simulink model "untitled"  (R2023b)
settings: Solver=VariableStepAuto  StartTime=0.0  StopTime=1  RelTol=1e-3
libraries: commdigbbndpm3 x2, dspfdesign x2, commchan3 x1, commsink2 x1, commrandsrc3 x1
settings Model: Creator=Bunakov Egor  LastModifiedBy=Bunakov Egor

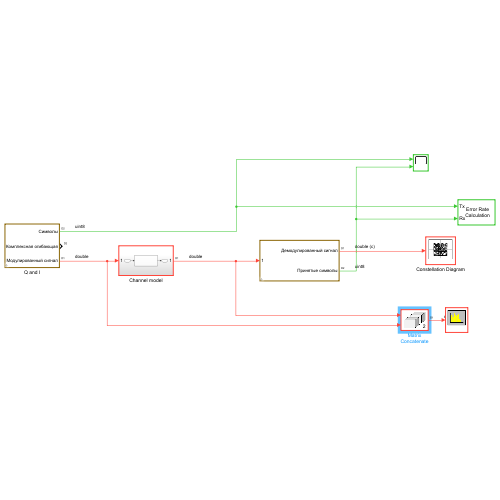
[thumbnail: Simulink's stored preview of the top-level diagram]
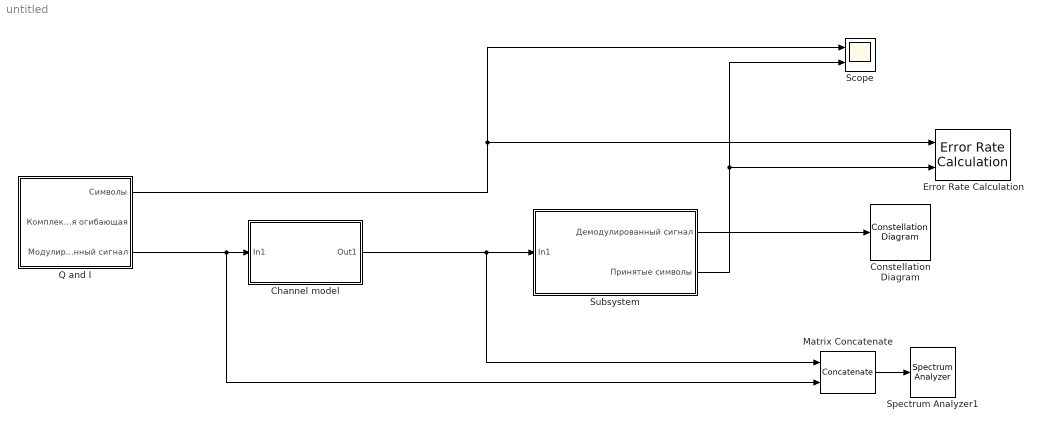
== system untitled ==
  Channel model : Subsystem
  Constellation Diagram : ConstellationDiagram  WindowPosition=[220.000000,9.000000,600.000000,600.000000,]  ScopeFrameLocation=window  ShowTrajectory=on
  Error Rate Calculation : commsink2/Error Rate Calculation  N=0  st_delay=0  cp_mode=Entire frame  subframe=[]  PMode=Workspace  WsName=ErrorVec  RsMode2=off  stop=off  numErr=100  maxBits=1e6
      settings: LibrarySourceBlock=|
      | commhdlsink/Error Rate
      | Calculation
  Matrix Concatenate : Concatenate  Mode=Multidimensional array  ConcatenateDimension=2
  Q and I : Subsystem  mask{CarrierFrequency=10000, SamplingFrequency=100000, SymbolRate=1000}
      mask prompts: CarrierFrequency "Частота несущей"; SamplingFrequency "Частота отрисовки синуса"; SymbolRate "Частота прихода данных"
  Scope : Scope  NumInputPorts=2
  Spectrum Analyzer1 : SpectrumAnalyzer  WindowPosition=[567.000000,192.000000,800.000000,500.000000,]  ScopeFrameLocation=window  YLimits=[-52.67376083,21.22078734]
  Subsystem : Subsystem  mask{SymbolRate=1000, CarrierFrequency=10000, SamplingFrequency=100000}
      mask prompts: SymbolRate "Частота выхода данных"; CarrierFrequency "Частота несущей"; SamplingFrequency "Частота отрисовки синуса"
  wires:
  Q and I/3(Модулированный сигнал) -> Matrix Concatenate/2, Channel model/1(In1)
  Channel model/1(Out1) -> Matrix Concatenate/1, Subsystem/1(In1)
  Subsystem/1(Демодулированный сигнал) -> Constellation Diagram/1
  Q and I/1(Символы) -> Error Rate Calculation/1, Scope/1
  Subsystem/2(Принятые символы) -> Error Rate Calculation/2, Scope/2
  Matrix Concatenate/1 -> Spectrum Analyzer1/1

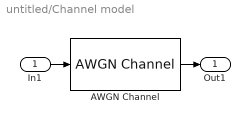
== system untitled/Channel model ==
  In1 : Inport
  AWGN Channel : commchan3/AWGN Channel  LegacyMode=off  NoiseMethod="Signal to noise ratio  (SNR)"  noiseMode="Signal to noise ratio  (SNR)"  EbNo=10  EsNo=10  SNR=100  BitsPerSymbol=1  SignalPower=1  SamplesPerSymbol=1  SymbolPeriod=1  VarianceSource=Parameter  Variance=1  RandomStream=Global stream  Seed=67  SimulateUsing=Code generation
  Out1 : Outport
  wires:
  In1/1 -> AWGN Channel/1
  AWGN Channel/1 -> Out1/1

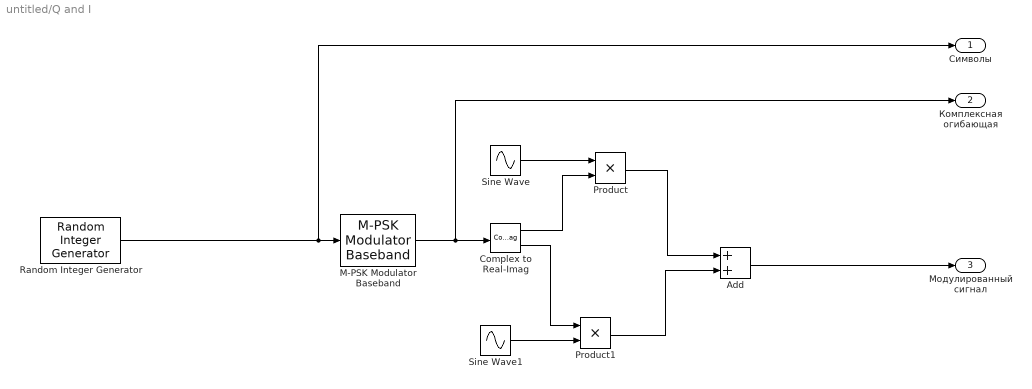
== system untitled/Q and I ==
  Add : Sum
  Complex to Real-Imag : ComplexToRealImag
  M-PSK Modulator Baseband : commdigbbndpm3/M-PSK Modulator Baseband  M=4  InType=Integer  Enc=Gray  Mapping=[0:7]  Ph=pi/4  outDtype=double  outWordLen=16  outUDDataType=sfix(16)  outFracLenMode=Best precision  outFracLen=15  outDataTypeStr=double  outLastDataTypeStr=double
      settings: LibrarySourceBlock=|
      | commhdldigbbndpm/M-PSK
      | Modulator
      | Baseband
  Product : Product
  Product1 : Product
  Random Integer Generator : commrandsrc3/Random Integer Generator  SetSize=4  SeedSource=Auto  Seed=0  SampleTime=1/SymbolRate  SamplesPerFrame=1  OutputDataType=uint8  SimulateUsing=Interpreted execution
  Sine Wave : Sin  Frequency=2*pi*CarrierFrequency  SampleTime=1/SamplingFrequency
  Sine Wave1 : Sin  Frequency=2*pi*CarrierFrequency  Phase=pi/2  SampleTime=1/SamplingFrequency
  Символы : Outport
  Комплексная огибающая : Outport  Port=2
  Модулированный сигнал : Outport  Port=3
  wires:
  Random Integer Generator/1 -> M-PSK Modulator Baseband/1, Символы/1
  M-PSK Modulator Baseband/1 -> Комплексная огибающая/1, Complex to Real-Imag/1
  Sine Wave/1 -> Product/1
  Complex to Real-Imag/1 -> Product/2
  Sine Wave1/1 -> Product1/2
  Complex to Real-Imag/2 -> Product1/1
  Product1/1 -> Add/2
  Product/1 -> Add/1
  Add/1 -> Модулированный сигнал/1

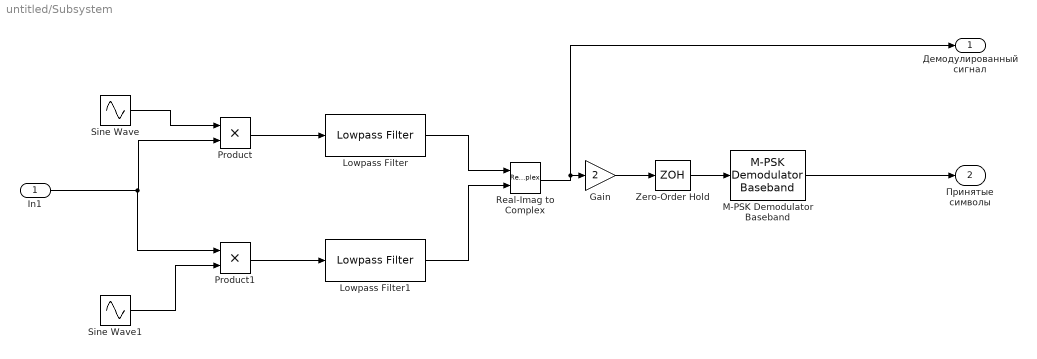
== system untitled/Subsystem ==
  In1 : Inport
  Gain : Gain  Gain=2
  Lowpass Filter : dspfdesign/Lowpass Filter  FilterType=FIR  DesignForMinimumOrder=on  FilterOrder=50  PassbandFrequency=CarrierFrequency  StopbandFrequency=CarrierFrequency*1.2  PassbandRipple=0.1  StopbandAttenuation=80  SampleRateMode=Specify on dialog  SampleRate=SamplingFrequency  SimulateUsing=Interpreted execution  roundingMode=Floor  coeffsDataTypeStr=fixdt(1,16)
  Lowpass Filter1 : dspfdesign/Lowpass Filter  FilterType=FIR  DesignForMinimumOrder=on  FilterOrder=50  PassbandFrequency=CarrierFrequency  StopbandFrequency=CarrierFrequency*1.2  PassbandRipple=0.1  StopbandAttenuation=80  SampleRateMode=Specify on dialog  SampleRate=SamplingFrequency  SimulateUsing=Interpreted execution  roundingMode=Floor  coeffsDataTypeStr=fixdt(1,16)
  M-PSK Demodulator Baseband : commdigbbndpm3/M-PSK Demodulator Baseband  M=4  OutType=Integer  DecType=Hard decision  VarSource=Dialog  Variance=1  Dec=Gray  Mapping=[0:7]  Ph=pi/4  outDtype1=Inherit via internal rule  outDtype2=Inherit via internal rule  derotateFactorWordLen=16  derotateFactorDataTypeStr=Inherit: Same word length as input  derotateFactorLastDataTypeStr=Inherit: Same word length as input
      settings: LibrarySourceBlock=|
      | commhdldigbbndpm/M-PSK
      | Demodulator
      | Baseband
  Product : Product
  Product1 : Product
  Real-Imag to Complex : RealImagToComplex
  Sine Wave : Sin  Frequency=2*pi*CarrierFrequency  SampleTime=1/SamplingFrequency
  Sine Wave1 : Sin  Frequency=2*pi*CarrierFrequency  Phase=pi/2  SampleTime=1/SamplingFrequency
  Zero-Order Hold : ZeroOrderHold  SampleTime=1/SymbolRate
  Демодулированный сигнал : Outport
  Принятые символы : Outport  Port=2
  wires:
  Real-Imag to Complex/1 -> Демодулированный сигнал/1, Gain/1
  In1/1 -> Product1/1, Product/2
  Sine Wave/1 -> Product/1
  Product/1 -> Lowpass Filter/1
  Product1/1 -> Lowpass Filter1/1
  Lowpass Filter/1 -> Real-Imag to Complex/1
  Lowpass Filter1/1 -> Real-Imag to Complex/2
  Sine Wave1/1 -> Product1/2
  Zero-Order Hold/1 -> M-PSK Demodulator Baseband/1
  Gain/1 -> Zero-Order Hold/1
  M-PSK Demodulator Baseband/1 -> Принятые символы/1
